simulink model "DC_Motor_Speed_Control"  (R2024a)
settings: Solver=VariableStepAuto  StartTime=0.0  StopTime=10  RelTol=1e-3
libraries: spsIdealSwitchLib x6, spsSeriesRLCBranchLib x6, spsDCVoltageSourceLib x4, spsDCMachineLib x2, sps_lib x1
settings Model: Creator=Asus  LastModifiedBy=Asus

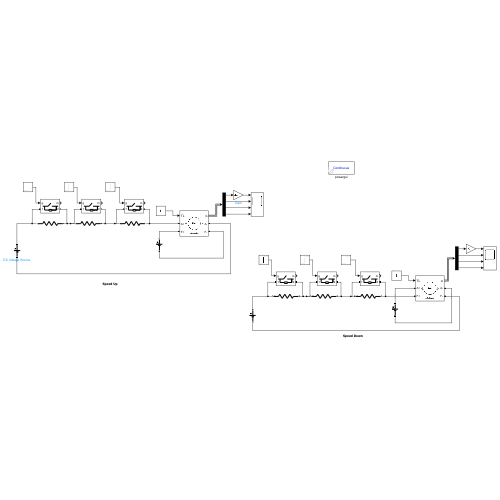
[thumbnail: Simulink's stored preview of the top-level diagram]
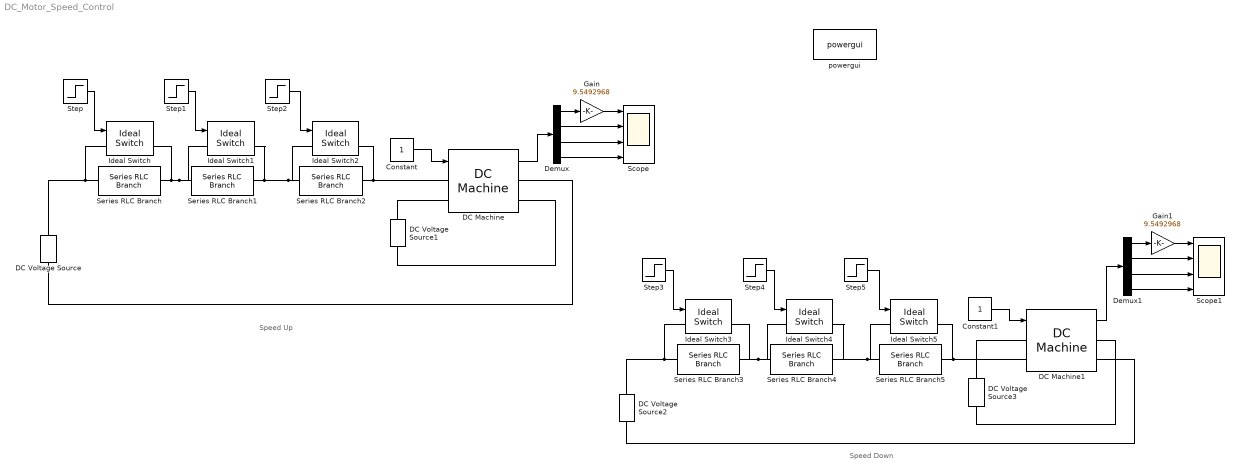
== system DC_Motor_Speed_Control ==
  note: Speed Up
  note: Speed Down
  Constant : Constant
  Constant1 : Constant
  DC Machine : spsDCMachineLib/DC Machine  PresetModel=01: 5HP 240V 1750RPM Field:300V  MechanicalLoad=Torque TL  FieldType=Wound  ShowDetailedParameters=on  MeasurementBus=off  RLa=[2.581 0.028]  RLf=[281.2 156]  Laf=0.9483  MachineConstant=Torque constant (N.m/A)  Ke=1.8  Kt=1.8  J=0.02215  Bm=0.002953  Tf=0.5161  w0=1  Ifinit=1.06685633001422  TsPowergui=0  TsBlock=-1
  DC Machine1 : spsDCMachineLib/DC Machine  PresetModel=01: 5HP 240V 1750RPM Field:300V  MechanicalLoad=Torque TL  FieldType=Wound  ShowDetailedParameters=on  MeasurementBus=off  RLa=[2.581 0.028]  RLf=[281.2 156]  Laf=0.9483  MachineConstant=Torque constant (N.m/A)  Ke=1.8  Kt=1.8  J=0.02215  Bm=0.002953  Tf=0.5161  w0=1  Ifinit=0.673814235988798  TsPowergui=0  TsBlock=-1
  DC Voltage Source : spsDCVoltageSourceLib/DC Voltage Source  Amplitude=240  Measurements=None
  DC Voltage Source1 : spsDCVoltageSourceLib/DC Voltage Source  Amplitude=300  Measurements=None
  DC Voltage Source2 : spsDCVoltageSourceLib/DC Voltage Source  Amplitude=240  Measurements=None
  DC Voltage Source3 : spsDCVoltageSourceLib/DC Voltage Source  Amplitude=300  Measurements=None
  Demux : Demux
  Demux1 : Demux
  Gain : Gain  Gain=9.5492968
  Gain1 : Gain  Gain=9.5492968
  Ideal Switch{,1..5} (6 alike) : spsIdealSwitchLib/Ideal Switch  Ron=0.001  Lon=0  IC=0  Rs=1e5  Cs=inf  Measurements=on
  Scope : Scope  NumInputPorts=4
  Scope1 : Scope  NumInputPorts=4
  Series RLC Branch{,1..5} (6 alike) : spsSeriesRLCBranchLib/Series RLC Branch  LConnTagsString=__new0  RConnTagsString=__new0  BranchType=R  Resistance=25  Inductance=1e-3  SetiL0=off  InitialCurrent=0  Capacitance=1e-6  Setx0=off  InitialVoltage=0  Measurements=None
  Step : Step  Time=2.5  SampleTime=0
  Step1 : Step  Time=5  SampleTime=0
  Step2 : Step  Time=7.5  SampleTime=0
  Step3 : Step  Time=2.5  SampleTime=0
  Step4 : Step  Time=5  SampleTime=0
  Step5 : Step  Time=7.5  SampleTime=0
  powergui : sps_lib/powergui  Priority=1  SimulationMode=Continuous  SampleTime=50e-6  frequency=60  Iterations=50  frequencyindice=0  Pbase=100e6  ErrMax=1e-4  UnitsV=kV  UnitsW=MW  buscounter=0  FunctionMessages=off  echomessages=off  EnableUseOfTLC=off  CurrentSourceSwitches=off  DisableSnubberDevices=off  DisableRonSwitches=off  DisableVfSwitches=off  DisplayEquations=off  AutomaticDiscreteSolvers=off  SolverType=Tustin/Backward Euler (TBE)  Interpol=off  ExternalGateDelay=off  methode=off  Ts=100  x0status=blocks  SPID=on  SwTol=0  HookPort=off  NonlinearTolerance=1e-4  nMaxIteration=100  ContinueOnMaxIteration=off  RestoreLinks=warning  ResistiveCurrentMeasurement=off  Frange=[0:2:500]  Ylog=off  Xlog=on  ShowGrid=off  save=off  variable=ZData  structure=0  ZoomFFT=off  StartTime=0.0  cycles=1  DisplayStyle=1  fundamental=60  FreqAxis=off  MaxFrequency=1000  frequencyindicesteady=1  RmsSteady=1  display=off
  wires:
  Constant/1 -> DC Machine/1
  DC Machine/1 -> Demux/1
  Demux/1 -> Gain/1
  Gain/1 -> Scope/1
  Demux/2 -> Scope/2
  Demux/3 -> Scope/3
  Demux/4 -> Scope/4
  Step/1 -> Ideal Switch/1
  Step1/1 -> Ideal Switch1/1
  Step2/1 -> Ideal Switch2/1
  Step5/1 -> Ideal Switch5/1
  Demux1/1 -> Gain1/1
  Demux1/3 -> Scope1/3
  Step4/1 -> Ideal Switch4/1
  Step3/1 -> Ideal Switch3/1
  Demux1/2 -> Scope1/2
  Demux1/4 -> Scope1/4
  DC Machine1/1 -> Demux1/1
  Gain1/1 -> Scope1/1
  Constant1/1 -> DC Machine1/1
  connections:
  DC Voltage Source/RConn1 -- Series RLC Branch/LConn1 -- Ideal Switch/LConn1
  DC Machine/RConn1 -- DC Voltage Source/LConn1
  DC Voltage Source1/RConn1 -- DC Machine/LConn2
  DC Voltage Source1/LConn1 -- DC Machine/RConn2
  Series RLC Branch/RConn1 -- Ideal Switch1/LConn1 -- Series RLC Branch1/LConn1 -- Ideal Switch/RConn1
  Series RLC Branch2/RConn1 -- Ideal Switch2/RConn1 -- DC Machine/LConn1
  Series RLC Branch1/RConn1 -- Ideal Switch2/LConn1 -- Series RLC Branch2/LConn1 -- Ideal Switch1/RConn1
  Series RLC Branch5/LConn1 -- Ideal Switch4/RConn1 -- Series RLC Branch4/RConn1 -- Ideal Switch5/LConn1
  Series RLC Branch4/LConn1 -- Ideal Switch3/RConn1 -- Series RLC Branch3/RConn1 -- Ideal Switch4/LConn1
  Series RLC Branch5/RConn1 -- Ideal Switch5/RConn1 -- DC Machine1/LConn2
  Ideal Switch3/LConn1 -- DC Voltage Source2/RConn1 -- Series RLC Branch3/LConn1
  DC Voltage Source3/RConn1 -- DC Machine1/LConn1
  DC Machine1/RConn1 -- DC Voltage Source3/LConn1
  DC Machine1/RConn2 -- DC Voltage Source2/LConn1
